simulink model "CdeRobot"  (R2016a)
settings: Solver=ode45  StartTime=0.0  StopTime=100.0  RelTol=1e-3
values from neighbouring files (symbols this model uses):
  Beff = 1/80    (= 0.0125)    [sf_loi_avant_RP_VERSION_ETUDIANT.m]    (also in test.m)
  Jeff = Jeff200    [test.m]
  K = K200    [sf_loi_avant_RP_VERSION_ETUDIANT.m]    (also in test.m)
  KD = KD200    [sf_loi_avant_RP_VERSION_ETUDIANT.m]    (also in test.m)
  Km_R = 0.3    [sf_loi_avant_RP_VERSION_ETUDIANT.m]    (also in test.m)
  r = R(1)    [sf_loi_avant_RP_VERSION_ETUDIANT.m]    (also in test.m)
libraries: simulink x2
settings Model: Creator=2asri13  LastModifiedBy=Ludwig
settings DataIOCC: LimitDataPoints=on  SaveFormat=Array
settings DebuggingCC: SolverPrmCheckMsg=warning
settings HardwareCC: ProdBitPerPointer=32  ProdLargestAtomicFloat=None  ProdIntDivRoundTo=Undefined  ProdEndianess=Unspecified  ProdWordSize=32  ProdHWDeviceType=32-bit Generic
settings ModelReferenceCC: PropagateSignalLabelsOutOfModel=off
settings ConfigComp: CovModelRefEnable=Off  CovSFcnEnable=off

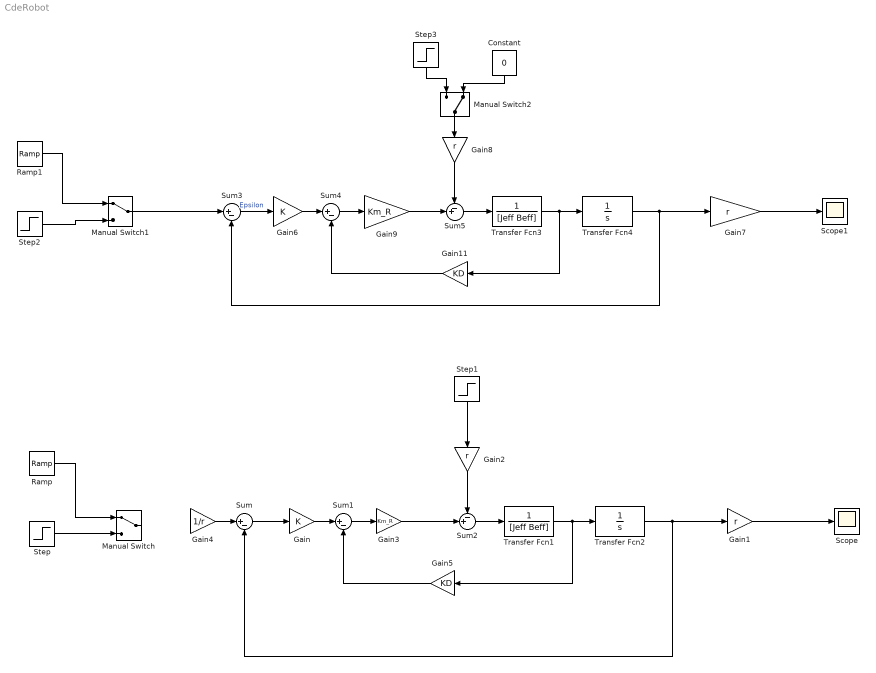
== system CdeRobot ==
  Constant : Constant  Value=0
  Gain : Gain  Gain=K
  Gain{1..2,7..8} (4 alike) : Gain  Gain=r
  Gain11 : Gain  Gain=KD
  Gain3 : Gain  Gain=Km_R
  Gain4 : Gain  Gain=1/r
  Gain5 : Gain  Gain=KD
  Gain6 : Gain  Gain=K
  Gain9 : Gain  Gain=Km_R
  Manual Switch : ManualSwitch
  Manual Switch1 : ManualSwitch
  Manual Switch2 : ManualSwitch  CurrentSetting=0
  Ramp : simulink/Sources/Ramp  slope=1  start=0  X0=0
  Ramp1 : simulink/Sources/Ramp  slope=1  start=0  X0=0
  Scope : Scope
  Scope1 : Scope
  Step : Step  Time=0  SampleTime=0
  Step1 : Step  After=10  SampleTime=0
  Step2 : Step  Time=0  SampleTime=0
  Step3 : Step  After=10  SampleTime=0
  Sum{,1,3..4} (4 alike) : Sum  Inputs=|+-
  Sum2 : Sum  Inputs=-+|
  Sum5 : Sum  Inputs=-+|
  Transfer Fcn1 : TransferFcn  Denominator=[Jeff Beff]
  Transfer Fcn2 : TransferFcn  Denominator=[1 0]
  Transfer Fcn3 : TransferFcn  Denominator=[Jeff Beff]
  Transfer Fcn4 : TransferFcn  Denominator=[1 0]
  wires:
  Sum/1 -> Gain/1
  Gain/1 -> Sum1/1
  Sum1/1 -> Gain3/1
  Gain3/1 -> Sum2/2
  Sum2/1 -> Transfer Fcn1/1
  Transfer Fcn1/1 -> Gain5/1, Transfer Fcn2/1
  Transfer Fcn2/1 -> Sum/2, Gain1/1
  Gain1/1 -> Scope/1
  Gain2/1 -> Sum2/1
  Step1/1 -> Gain2/1
  Gain4/1 -> Sum/1
  Gain5/1 -> Sum1/2
  Ramp/1 -> Manual Switch/1
  Step/1 -> Manual Switch/2
  Sum3/1 -> Gain6/1  "Epsilon"
  Gain6/1 -> Sum4/1
  Sum4/1 -> Gain9/1
  Gain9/1 -> Sum5/2
  Sum5/1 -> Transfer Fcn3/1
  Transfer Fcn3/1 -> Gain11/1, Transfer Fcn4/1
  Transfer Fcn4/1 -> Sum3/2, Gain7/1
  Gain7/1 -> Scope1/1
  Gain8/1 -> Sum5/1
  Manual Switch1/1 -> Sum3/1
  Gain11/1 -> Sum4/2
  Ramp1/1 -> Manual Switch1/1
  Step2/1 -> Manual Switch1/2
  Manual Switch2/1 -> Gain8/1
  Step3/1 -> Manual Switch2/1
  Constant/1 -> Manual Switch2/2
